simulink model "ringmod"  (R2014b)
settings: Solver=ode45  StartTime=0.0  StopTime=10.0  RelTol=1e-3
libraries: dspvision x1, dspsnks4 x1
settings Model: Creator=ICLab  LastModifiedBy=ICLab
settings OptimizationCC: OptimizeModelRefInitCode=on  LifeSpan=1
settings RTWCC: SystemTargetFile=ert.tlc  TemplateMakefile=ert_default_tmf  Description=Embedded Coder  ProcessScript=ert_make_rtw_hook
settings CodeAppCC: IgnoreCustomStorageClasses=off
settings ERTTargetCC: CodeReplacementLibrary=ARM Cortex-M  GenerateSampleERTMain=on  ERTCustomFileTemplate=example_file_process.tlc

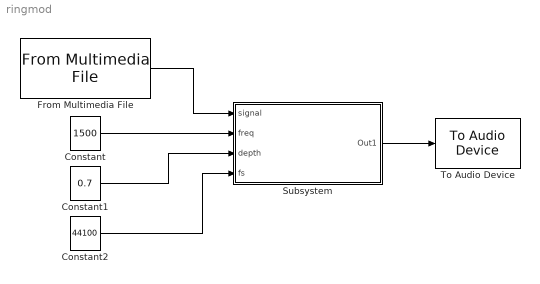
== system ringmod ==
  Constant : Constant  Value=1500  VectorParams1D=off
  Constant1 : Constant  Value=0.7  VectorParams1D=off
  Constant2 : Constant  Value=44100  VectorParams1D=off
  From Multimedia File : dspvision/From Multimedia File  inputFilename=C:\Users\ICLab\Desktop\Embedded system\MATLAB_DSP\ringmod\deltaclick.wav  loop=on  numPlays=inf  outputStreams=Audio only  videoDataType=single  audioDataType=double  inheritSampleTime=on  userDefinedSampleTime=1/30  noAudioOutput=off  isIntensityVideo=off  fourcc=RGB  colorVideoFormat=Separate color signals  outputEOF=off  dataOrg=Column-major  audioFrameSize=1024  computeAudioFrameSize=off  outSamplingMode=Frame based
  Subsystem : Subsystem
  To Audio Device : dspsnks4/To Audio Device  deviceName=Default  inheritSampleRate=on  sampleRate=44100  deviceDatatype=Determine from input data type  autoBufferSize=on  bufferSize=4096  queueDuration=1.0  defaultOutputChannelMapping=on  outputChannelMapping=1:2  outputNumUnderrunSamples=off
  wires:
  Subsystem/1(Out1) -> To Audio Device/1
  From Multimedia File/1 -> Subsystem/1(signal)
  Constant/1 -> Subsystem/2(freq)
  Constant1/1 -> Subsystem/3(depth)
  Constant2/1 -> Subsystem/4(fs)

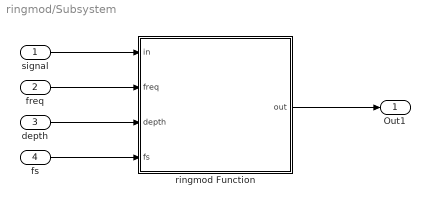
== system ringmod/Subsystem ==
  signal : Inport
  freq : Inport  Port=2
  depth : Inport  Port=3
  fs : Inport  Port=4
  ringmod Function : MATLAB Function  TreatAsAtomicUnit=on
  Out1 : Outport
  wires:
  signal/1 -> ringmod Function/1(in)
  freq/1 -> ringmod Function/2(freq)
  depth/1 -> ringmod Function/3(depth)
  fs/1 -> ringmod Function/4(fs)
  ringmod Function/1(out) -> Out1/1

== matlab function ringmod/Subsystem/ringmod Function ==
  data: in input; out output; freq input; depth input; fs input
function out   = ringmod( in, freq, depth, fs )
%RINGMOD ring modulates input signal at specified frequency and depth
% in is input signal
% modfreq is frequency of the ring mod
% depth ranges 0 (no ringmod added) to 1 (equal amplitude added)
% fs is sampling freq of input signal

n = (1:length(in))';
wave = depth*sin(2*pi*freq/fs .*n);
modulated = wave.*in;

out = in + modulated;

end
